simulink model "Two_Node"  (R2022b)
settings: Solver=VariableStepAuto  StartTime=0.0  StopTime=300  RelTol=1e-3
model workspace (MATLAB code in the model file):
  | J_M=7;
  | K_1=3;
  | K_1d=15;
  | KM=2;
  | K_3=2;
  | K_4=1;
  | K_5=10^-7;
  | x_star(1)=K_4/K_3;
  | x_star(2)=J_M*K_1/(K_1d*x_star(1)/(KM+x_star(1)))-K_1;
values from neighbouring files (symbols this model uses):
  x_star = [0.4;0.64;0.5]    [node3IFFN.m]    (also in node3NFB2.m; node3NFB3.m; node5IFF.m = [0.1875; 0.250; 0.5000; 0.8000; 0.3125]; node5IFF2.m = [0.1875; 0.250; 0.5000; 0.8000; 0.3125])
settings Model: Creator=pxb271  LastModifiedBy=pxb271

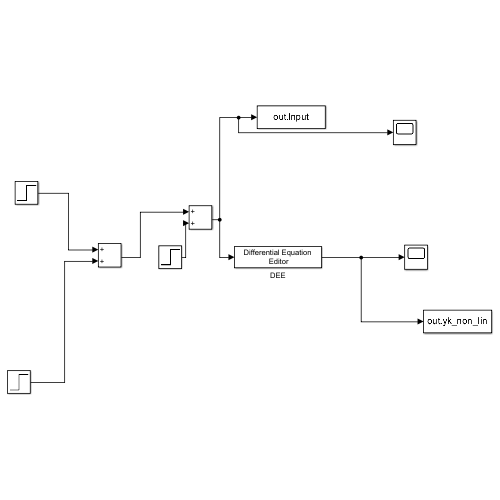
[thumbnail: Simulink's stored preview of the top-level diagram]
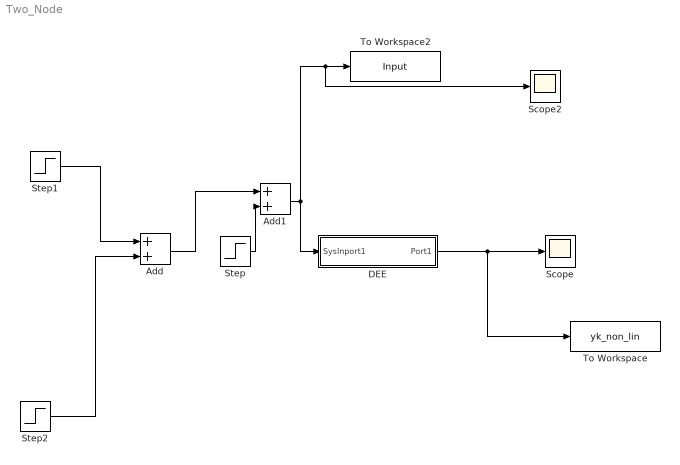
== system Two_Node ==
  Add : Sum
  Add1 : Sum
  DEE : Subsystem  mask(Differential Equation Editor (DEE)){}
      settings: OpenFcn=diffeqed
      mask Display: disp('Differential Equation\n Editor')
  Scope : Scope
  Scope2 : Scope
  Step : Step  Time=200  After=0.15  SampleTime=0
  Step1 : Step  Time=5  SampleTime=0
  Step2 : Step  Time=100  After=0.2  SampleTime=0
  To Workspace : ToWorkspace  VariableName=yk_non_lin  SampleTime=-1
  To Workspace2 : ToWorkspace  VariableName=Input  SampleTime=-1
  wires:
  Add/1 -> Add1/1
  Step/1 -> Add1/2
  Step1/1 -> Add/1
  DEE/1(Port1) -> To Workspace/1, Scope/1
  Step2/1 -> Add/2
  Add1/1 -> DEE/1(SysInport1), Scope2/1, To Workspace2/1

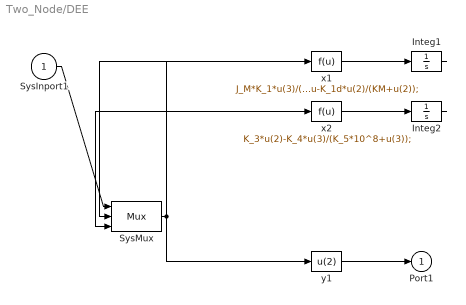
== system Two_Node/DEE ==
  SysInport1 : Inport
  Integ1 : Integrator  InitialCondition=x_star(1)
  Integ2 : Integrator  InitialCondition=x_star(2)
  SysMux : Mux  Inputs=3
  x1 : Fcn  Expr=J_M*K_1*u(3)/(K_1+u(3))+u-K_1d*u(2)/(KM+u(2));
  x2 : Fcn  Expr=K_3*u(2)-K_4*u(3)/(K_5*10^8+u(3));
  y1 : Fcn  Expr=u(2)
  Port1 : Outport
  wires:
  SysInport1/1 -> SysMux/1
  SysMux/1 -> x1/1, x2/1, y1/1
  x1/1 -> Integ1/1
  Integ1/1 -> SysMux/2
  x2/1 -> Integ2/1
  Integ2/1 -> SysMux/3
  y1/1 -> Port1/1
